simulink library "anngaincalc"  (R2022b)
settings: Solver=VariableStepAuto  StartTime=0.0  StopTime=10.0  RelTol=1e-3
undefined symbols (not defined in the file or in its folder): Fs, L, nAnnIn
libraries: AnnGainCalcBtc x1
settings Model: Creator=nikunj.tapodhan  LastModifiedBy=kl13806
settings SolverCC: AlgebraicLoopSolver=TrustRegion
settings DebuggingCC: UnconnectedInputMsg=warning  UnconnectedOutputMsg=warning  UnconnectedLineMsg=warning  SFMachineParentedDataDiag=warning  ArithmeticOperatorsInVariantConditions=warning
settings ModelReferenceCC: EnableRefExpFcnMdlSchedulingChecks=on
settings SFSimCC: CustomCodeUndefinedFunction=UseInterfaceOnly
settings RTWCC: DLArmComputeVersion=19.05

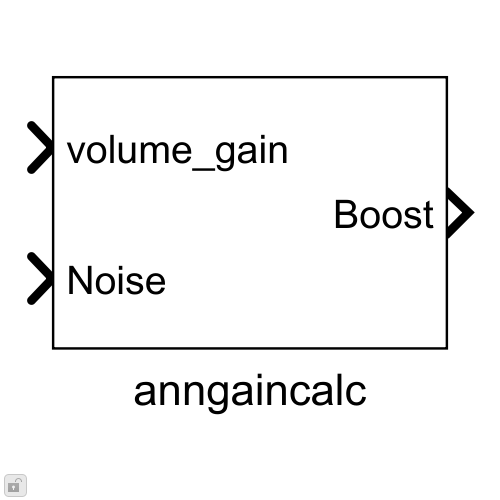
[thumbnail: Simulink's stored preview of the top-level diagram]
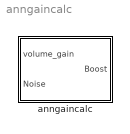
== system anngaincalc ==
  anngaincalc : Subsystem  mask{vncEnable=1, vncBoostGain=1, VNCThresh=zeros(1,nAnnIn), VNCSlope=0.4.*ones(1,nAnnIn), maxBoost=18.*ones(1,nAnnIn), maxSPL=120.*ones(1,nAnnIn), minVNCSignal=40, rampTau=0.1, rampCoef=0, Fd=Fs/L, NoiseOverRideFlag=0, NoiseOverRide=0, boostOverRideFlag=zeros(1,nAnnIn), boostOverRide=zeros(1,nAnnIn)}
      mask prompts: vncEnable "vnc Enable"; vncBoostGain "vnc Boost Gain"; VNCThresh "VNC Threshold"; VNCSlope "VNC Slope"; maxBoost "Max Boost"; maxSPL "Max SPL"; minVNCSignal "Min VNC Signal"; rampTau "Ramp Tau"; rampCoef "Ramp Coefficients"; Fd "Decimated Rate (Fd)"; NoiseOverRideFlag "Noise OverRide Flag"; NoiseOverRide "Noise OverRide Value"; boostOverRideFlag "Boost OverRide Flag"; boostOverRide "Boost OverRide Value"
      mask init:
      | blkh = gcbh;
      | % Copy discrete mask parameters into a classdef object
      | InnerLinkConfig = AnnGainCalcConfig;
      | InnerLinkConfig.VncEnable = vncEnable;
      | InnerLinkConfig.VncBoostGain = vncBoostGain;
      | InnerLinkConfig.VncThresh = VNCThresh;
      | InnerLinkConfig.VncSlope = VNCSlope;
      | InnerLinkConfig.MaxBoost = maxBoost;
      | InnerLinkConfig.MaxSpl = maxSPL;
      | InnerLinkConfig.MinVncSignal = minVNCSignal;
      | InnerLinkConfig.RampTau = rampTau;
      | % InnerLinkConfig.RampCoef = rampCoef;
      | InnerLinkConfig.Fd = Fd;
      | InnerLinkConfig.NoiseOverrideFlag = NoiseOverRideFlag;
      | InnerLinkConfig.NoiseOverride = NoiseOverRide;
      | InnerLinkConfig.BoostOverrideFlag = boostOverRideFlag;
      | InnerLinkConfig.BoostOverride = boostOverRide;
      mask DialogControl ParameterGroupVar2 Prompt: OverRides

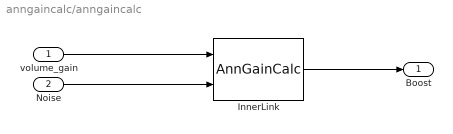
== system anngaincalc/anngaincalc ==
  volume_gain : Inport
  Noise : Inport  Port=2
  InnerLink : AnnGainCalcBtc/AnnGainCalc  Config=InnerLinkConfig  FeatureName=gaincalc
      settings: SourceProductName=Bose Blocklib
  Boost : Outport
  wires:
  volume_gain/1 -> InnerLink/1
  Noise/1 -> InnerLink/2
  InnerLink/1 -> Boost/1
